simulink model "hw2_q3_part_one"  (R2022b)
settings: Solver=ode4  StartTime=0.0  StopTime=10.0  FixedStep=0.001  RelTol=1e-3
settings Model: Creator=gaura  LastModifiedBy=gaura

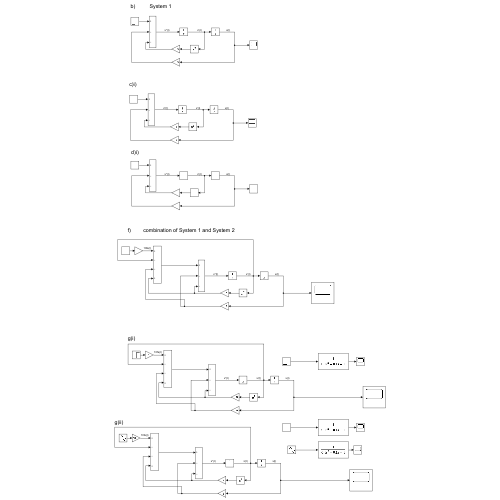
[thumbnail: Simulink's stored preview of the top-level diagram]
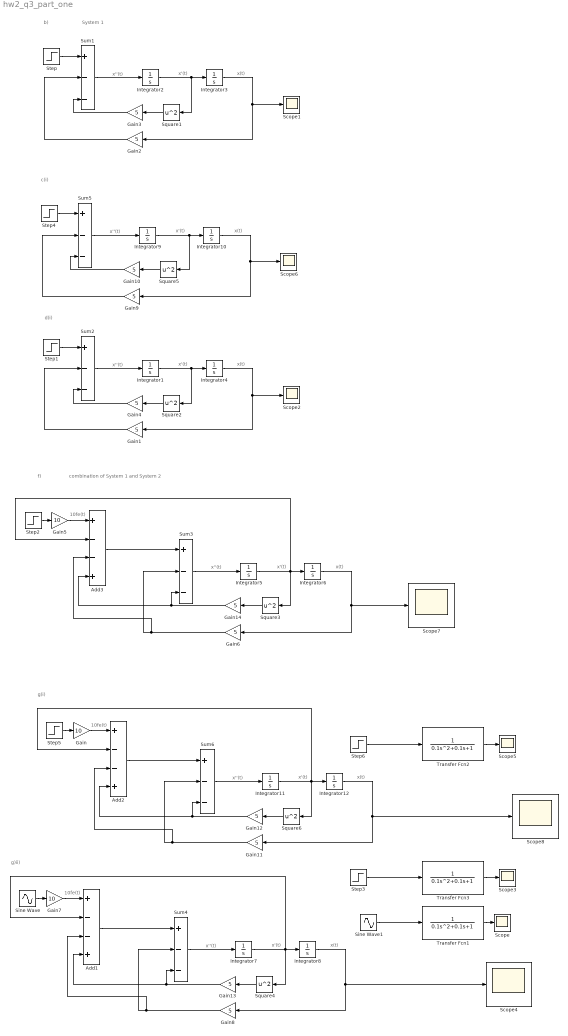
== system hw2_q3_part_one ==
  note: 10fe(t)
  note: System 1
  note: f)
  note: x(t)
  note: x''(t)
  note: x'(t)
  note: x'(t)
  note: x''(t)
  note: x(t)
  note: d)i)
  note: b)
  note: c)i)
  note: x(t)
  note: x''(t)
  note: x'(t)
  note: combination of System 1 and System 2
  note: x'(t)
  note: x(t)
  note: x''(t)
  note: g)i)
  note: 10fe(t)
  note: x'(t)
  note: x(t)
  note: g)ii)
  note: x''(t)
  note: 10fe(t)
  note: x'(t)
  note: x(t)
  note: x''(t)
  Add1 : Sum  Inputs=+--+
  Add2 : Sum  Inputs=+--+
  Add3 : Sum  Inputs=+--+
  Gain : Gain  Gain=10
  Gain{1..4,6,8..14} (12 alike) : Gain  Gain=5
  Gain5 : Gain  Gain=10
  Gain7 : Gain  Gain=10
  Integrator{1..12} (12 alike) : Integrator
  Scope{,1..8} (9 alike) : Scope
  Sine Wave : Sin  Frequency=3  SampleTime=0
  Sine Wave1 : Sin  Frequency=3  SampleTime=0
  Square{1..6} (6 alike) : Math  Operator=square
  Step{,2..6} (6 alike) : Step  Time=0  SampleTime=0
  Step1 : Step  Time=0  After=2  SampleTime=0
  Sum{1..6} (6 alike) : Sum  Inputs=+--
  Transfer Fcn1 : TransferFcn  Denominator=[0.1 0.1 1]
  Transfer Fcn2 : TransferFcn  Denominator=[0.1 0.1 1]
  Transfer Fcn3 : TransferFcn  Denominator=[0.1 0.1 1]
  wires:
  Gain2/1 -> Sum1/2
  Integrator3/1 -> Gain2/1, Scope1/1
  Integrator2/1 -> Square1/1, Integrator3/1
  Gain3/1 -> Sum1/3
  Step/1 -> Sum1/1
  Square1/1 -> Gain3/1
  Sum1/1 -> Integrator2/1
  Step1/1 -> Sum2/1
  Gain1/1 -> Sum2/2
  Integrator1/1 -> Square2/1, Integrator4/1
  Integrator4/1 -> Gain1/1, Scope2/1
  Sum2/1 -> Integrator1/1
  Square2/1 -> Gain4/1
  Gain4/1 -> Sum2/3
  Gain10/1 -> Sum5/3
  Sum5/1 -> Integrator9/1
  Gain9/1 -> Sum5/2
  Integrator10/1 -> Gain9/1, Scope6/1
  Step4/1 -> Sum5/1
  Integrator9/1 -> Square5/1, Integrator10/1
  Square5/1 -> Gain10/1
  Integrator12/1 -> Gain11/1, Scope8/1
  Gain12/1 -> Add2/4, Sum6/3
  Step5/1 -> Gain/1
  Integrator11/1 -> Add2/2, Square6/1, Integrator12/1
  Add2/1 -> Sum6/1
  Sum6/1 -> Integrator11/1
  Gain11/1 -> Add2/3, Sum6/2
  Square6/1 -> Gain12/1
  Gain/1 -> Add2/1
  Gain7/1 -> Add1/1
  Sine Wave/1 -> Gain7/1
  Square4/1 -> Gain13/1
  Gain8/1 -> Add1/3, Sum4/2
  Add1/1 -> Sum4/1
  Gain13/1 -> Add1/4, Sum4/3
  Integrator7/1 -> Add1/2, Square4/1, Integrator8/1
  Sum4/1 -> Integrator7/1
  Integrator8/1 -> Gain8/1, Scope4/1
  Sine Wave1/1 -> Transfer Fcn1/1
  Transfer Fcn1/1 -> Scope/1
  Transfer Fcn2/1 -> Scope5/1
  Step6/1 -> Transfer Fcn2/1
  Gain5/1 -> Add3/1
  Step2/1 -> Gain5/1
  Square3/1 -> Gain14/1
  Gain6/1 -> Add3/3, Sum3/2
  Add3/1 -> Sum3/1
  Integrator5/1 -> Add3/2, Square3/1, Integrator6/1
  Sum3/1 -> Integrator5/1
  Integrator6/1 -> Gain6/1, Scope7/1
  Gain14/1 -> Add3/4, Sum3/3
  Transfer Fcn3/1 -> Scope3/1
  Step3/1 -> Transfer Fcn3/1
